simulink model "FWMAV_DirectDrive"  (R2026a)
settings: Solver=ode4  StopTime=tStop  FixedStep=1e-5  MaxStep=1e-4  RelTol=1e-5  AbsTol=1e-7
values from neighbouring files (symbols this model uses):
  airDensity = 1.225    [FWMAV_Setup.m]
  alphaCoeff = 5e-3    (= 0.005)    [FWMAV_Setup.m]
  bm = bmRaw  * gearRatio^2    (= 3.6e-06)    [FWMAV_Setup.m]
  driveOmega = 2*pi*driveFreq    [FWMAV_FrequencySweep.m]    (also in FWMAV_Setup.m; FWMAV_SimulateInner.m = 2*pi*designFreq)
  driveVoltage = ratedVoltage    (= 3)    [FWMAV_Setup.m]
  hubLength = 0.01    [FWMAV_Setup.m]    (also in FWMAV_SimulateInner.m = params.hubLength)
  Jtotal = Jm + Jw + jAddedMass    [FWMAV_Setup.m]    (also in FWMAV_SimulateInner.m = params.Jm + Jw + jAddedMass)
  Kb = KbRaw * gearRatio    (= 0.01)    [FWMAV_Setup.m]
  kSpring = 0.01580    (= 0.0158)    [FWMAV_Setup.m]
  Kt = KtRaw * gearRatio * gearEfficiency    (= 0.01)    [FWMAV_Setup.m]
  La = 29e-3    (= 0.029)    [FWMAV_Setup.m]
  omegaSmooth = 1.0    (= 1)    [FWMAV_Setup.m]
  Ra = 9    [FWMAV_Setup.m]
  rootChord = wingLength / aspectRatio    (= 0.0201633333333)    [FWMAV_Setup.m]    (also in FWMAV_SimulateInner.m = designLw / params.aspectRatio)
  tauCoulomb = 0.00    (= 0)    [FWMAV_Setup.m]
  wingLength = 0.06049    [FWMAV_Setup.m]
settings Model: Creator=Saatvik  LastModifiedBy=Saatvik

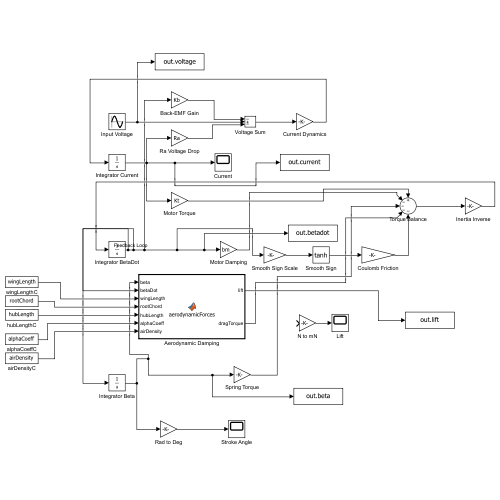
[thumbnail: Simulink's stored preview of the top-level diagram]
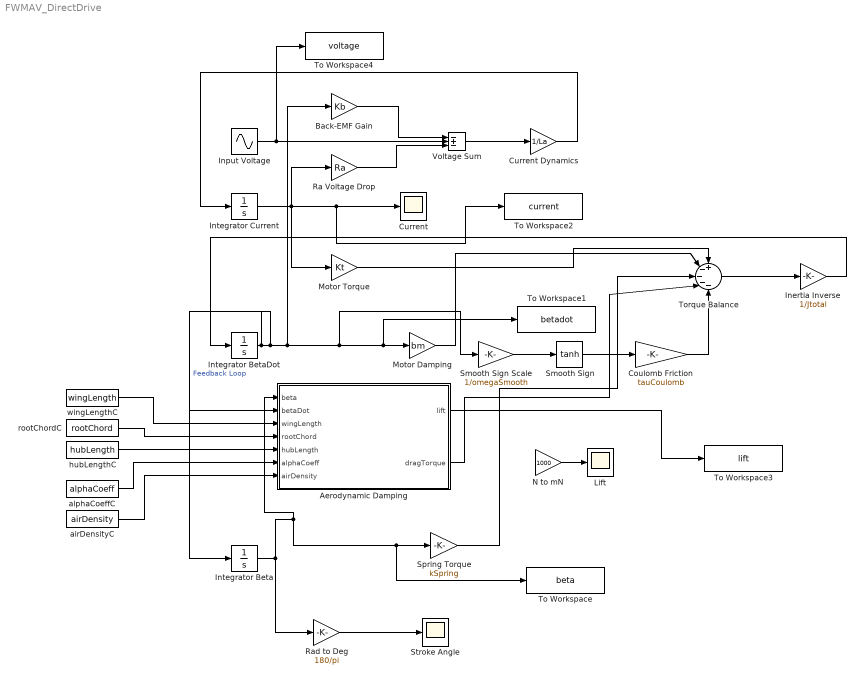
== system FWMAV_DirectDrive ==
  Aerodynamic Damping : MATLAB Function  TreatAsAtomicUnit=on
  Back-EMF Gain : Gain  Gain=Kb
  Coulomb Friction : Gain  Gain=tauCoulomb
  Current : Scope
      settings: ActiveDisplayYMinimum=-1.20668  ActiveDisplayYMaximum=0.80064  DataLoggingVariableName=ScopeData2
  Current Dynamics : Gain  Gain=1/La
  Inertia Inverse : Gain  Gain=1/Jtotal
  Input Voltage : Sin  Amplitude=driveVoltage  Frequency=driveOmega  SampleTime=0
  Integrator Beta : Integrator
  Integrator BetaDot : Integrator
  Integrator Current : Integrator
  Lift : Scope
      settings: ActiveDisplayYMinimum=-14.63039  ActiveDisplayYMaximum=131.67355
  Motor Damping : Gain  Gain=bm
  Motor Torque : Gain  Gain=Kt
  N to mN : Gain  Gain=1000
  Ra Voltage Drop : Gain  Gain=Ra
  Rad to Deg : Gain  Gain=180/pi
  Smooth Sign : Trigonometry  Operator=tanh
  Smooth Sign Scale : Gain  Gain=1/omegaSmooth
  Spring Torque : Gain  Gain=kSpring
  Stroke Angle : Scope
      settings: ActiveDisplayYMinimum=-116.0392  ActiveDisplayYMaximum=116.41251
  To Workspace : ToWorkspace  VariableName=beta  SaveFormat=Structure With Time  SampleTime=-1
  To Workspace1 : ToWorkspace  VariableName=betadot  SaveFormat=Structure With Time  SampleTime=-1
  To Workspace2 : ToWorkspace  VariableName=current  SaveFormat=Structure With Time  SampleTime=-1
  To Workspace3 : ToWorkspace  VariableName=lift  SaveFormat=Structure With Time  SampleTime=-1
  To Workspace4 : ToWorkspace  VariableName=voltage  SaveFormat=Structure With Time  SampleTime=-1
  Torque Balance : Sum  Inputs=+----
  Voltage Sum : Sum  Inputs=-+-
  airDensityC : Constant  Value=airDensity
  alphaCoeffC : Constant  Value=alphaCoeff
  hubLengthC : Constant  Value=hubLength
  rootChordC : Constant  Value=rootChord
  wingLengthC : Constant  Value=wingLength
  wires:
  Input Voltage/1 -> To Workspace4/1, Voltage Sum/2
  Ra Voltage Drop/1 -> Voltage Sum/3
  Back-EMF Gain/1 -> Voltage Sum/1
  Voltage Sum/1 -> Current Dynamics/1
  Current Dynamics/1 -> Integrator Current/1
  Integrator Current/1 -> To Workspace2/1, Current/1, Motor Torque/1, Ra Voltage Drop/1
  Motor Torque/1 -> Torque Balance/1
  Integrator BetaDot/1 -> Motor Damping/1, To Workspace1/1, Smooth Sign Scale/1, Back-EMF Gain/1, Integrator Beta/1, Aerodynamic Damping/2(betaDot)  "Feedback Loop"
  Motor Damping/1 -> Torque Balance/2
  Integrator Beta/1 -> To Workspace/1, Spring Torque/1, Aerodynamic Damping/1(beta), Rad to Deg/1
  Spring Torque/1 -> Torque Balance/3
  Torque Balance/1 -> Inertia Inverse/1
  Inertia Inverse/1 -> Integrator BetaDot/1
  Rad to Deg/1 -> Stroke Angle/1
  N to mN/1 -> Lift/1
  Aerodynamic Damping/2(dragTorque) -> Torque Balance/4
  Smooth Sign/1 -> Coulomb Friction/1
  Coulomb Friction/1 -> Torque Balance/5
  wingLengthC/1 -> Aerodynamic Damping/3(wingLength)
  rootChordC/1 -> Aerodynamic Damping/4(rootChord)
  hubLengthC/1 -> Aerodynamic Damping/5(hubLength)
  alphaCoeffC/1 -> Aerodynamic Damping/6(alphaCoeff)
  airDensityC/1 -> Aerodynamic Damping/7(airDensity)
  Smooth Sign Scale/1 -> Smooth Sign/1
  Aerodynamic Damping/1(lift) -> To Workspace3/1

== matlab function FWMAV_DirectDrive/Aerodynamic Damping ==
  data: beta input; betaDot input; lift output; dragTorque output; wingLength input; rootChord input; hubLength input; alphaCoeff input; airDensity input
function [lift, dragTorque] = aerodynamicForces(beta, betaDot, wingLength, rootChord, hubLength, alphaCoeff, airDensity)
%#codegen
    % Quasi-steady blade-element model with rotational drag.
    % Translational lift/drag from Sane-Dickinson 2002 fits.
    % Rotational drag added per Whitney & Wood 2010 (provides pitch-axis dissipation).
    % Added-mass is handled as a virtual inertia in FWMAV_Setup (constant offset on Jtotal).

    % Effective AoA from passive wing rotation
    alpha = pi/2 - alphaCoeff * abs(betaDot);
    if alpha < pi/4
        alpha = pi/4;
    end

    % Translational lift and drag coefficients (Sane-Dickinson 2002)
    cl = 0.225 + 1.58 * sin(2.13 * alpha - 0.1257);
    cd = 1.92  - 1.55 * cos(2.04 * alpha - 0.1714);

    % Rotational drag coefficient (Whitney & Wood 2010)
    cdRot = 5.0;

    % Blade-element integration along the span
    nElements = 100;
    rRoot = hubLength / 2;
    rTip  = wingLength + rRoot;
    dr = (rTip - rRoot) / (nElements - 1);

    liftSum = 0;
    dragTransSum = 0;
    dragRotSum = 0;
    halfRho = 0.5 * airDensity;

    for k = 1:nElements
        r = rRoot + (k - 1) * dr;
        chordRatio = (r - rRoot) / wingLength;
        chord = rootChord * sqrt(max(0.0, 1.0 - chordRatio^2));
        dArea = chord * dr;
        velSq = (r * betaDot)^2;

        liftSum       = liftSum       + halfRho * velSq * dArea * cl;
        dragTransSum  = dragTransSum  + halfRho * velSq * dArea * cd * r;
        % Rotational drag torque per element: 0.5*rho*cdRot*c^4 * betaDot*|betaDot| / 8
        dragRotSum    = dragRotSum    + cdRot * halfRho * chord^4 * dr / 8;
    end

    lift = liftSum;
    % Drag torque opposes motion in both directions
    dragTrans = dragTransSum;
    if betaDot < 0
        dragTrans = -dragTrans;
    end
    dragRot = dragRotSum * betaDot * abs(betaDot);
    dragTorque = dragTrans + dragRot;
end
